simulink model "siento"  (Simulink 7.2)
settings: Solver=ode45  StartTime=0.0  StopTime=10000.0  RelTol=1e-3
undefined symbols (not defined in the file or in its folder): aubt_proxy_ecg, aubt_proxy_emg, aubt_proxy_sc, ecgGen, FisherProjectionDisplay
libraries: dspbuff3 x4, simulink x1
settings Model: Creator=rafa  LastModifiedBy=rafa

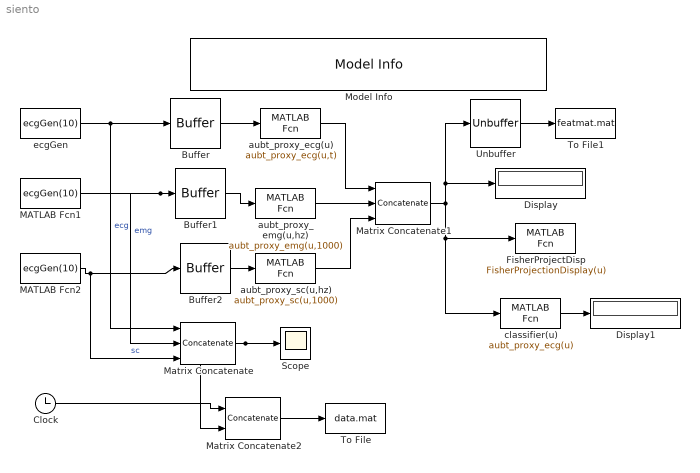
== system siento ==
  Buffer : dspbuff3/Buffer  N=10  V=0  ic=0
  Buffer1 : dspbuff3/Buffer  N=10  V=0  ic=0
  Buffer2 : dspbuff3/Buffer  N=10  V=0  ic=0
  Clock : Clock
      settings: Decimation=10
  Display : Display
  Display1 : Display
  FisherProjectDisp : MATLABFcn  MATLABFcn=FisherProjectionDisplay(u)  OutputDimensions=0
  MATLAB Fcn1 : MATLABFcn  MATLABFcn=ecgGen(10)
  MATLAB Fcn2 : MATLABFcn  MATLABFcn=ecgGen(10)
  Matrix Concatenate : Concatenate  NumInputs=3  Mode=Multidimensional array  ConcatenateDimension=2
  Matrix Concatenate1 : Concatenate  NumInputs=3  Mode=Multidimensional array  ConcatenateDimension=2
  Matrix Concatenate2 : Concatenate  Mode=Multidimensional array  ConcatenateDimension=2
  Model Info : simulink/Model-Wide Utilities/Model Info  SystemSampleTime=-1  InitialBlockCM=None  BlockCM=None  Frame=on  DisplayStringWithTags=|  HorizontalTextAlignment=Center  LeftAlignmentValue=0.5  SourceBlockDiagram=siento  TagMaxNumber=20
      | Siento Signal Processing
      | %<Description>First try
      | Last modified on %<LastModificationDate> (local time) by  %<LastModifiedBy>
  Scope : Scope
      settings: TimeRange=256  YMin=-1  YMax=1
  To File : ToFile  Filename=data.mat
  To File1 : ToFile  Filename=featmat.mat
  Unbuffer : dspbuff3/Unbuffer  ic=0
  aubt_proxy_ecg(u) : MATLABFcn  MATLABFcn=aubt_proxy_ecg(u,t)  OutputDimensions=1  Output1D=off
  aubt_proxy_emg(u,hz) : MATLABFcn  MATLABFcn=aubt_proxy_emg(u,1000)  OutputDimensions=1
  aubt_proxy_sc(u,hz) : MATLABFcn  MATLABFcn=aubt_proxy_sc(u,1000)  OutputDimensions=1
  classifier(u) : MATLABFcn  MATLABFcn=aubt_proxy_ecg(u)  OutputDimensions=1
  ecgGen : MATLABFcn  MATLABFcn=ecgGen(10)
  wires:
  ecgGen/1 -> Matrix Concatenate/1, Buffer/1  "ecg"
  MATLAB Fcn1/1 -> Matrix Concatenate/2, Buffer1/1  "emg"
  MATLAB Fcn2/1 -> Matrix Concatenate/3, Buffer2/1  "sc"
  Matrix Concatenate/1 -> Matrix Concatenate2/2, Scope/1
  aubt_proxy_ecg(u)/1 -> Matrix Concatenate1/1
  aubt_proxy_emg(u,hz)/1 -> Matrix Concatenate1/2
  aubt_proxy_sc(u,hz)/1 -> Matrix Concatenate1/3
  Matrix Concatenate1/1 -> Display/1, Unbuffer/1, classifier(u)/1, FisherProjectDisp/1
  classifier(u)/1 -> Display1/1
  Clock/1 -> Matrix Concatenate2/1
  Matrix Concatenate2/1 -> To File/1
  Buffer/1 -> aubt_proxy_ecg(u)/1
  Buffer1/1 -> aubt_proxy_emg(u,hz)/1
  Buffer2/1 -> aubt_proxy_sc(u,hz)/1
  Unbuffer/1 -> To File1/1
